simulink model "lyskawaProject_si"  (R2023b)
settings: Solver=VariableStepAuto  StartTime=startTime  StopTime=stopTime  MaxStep=maxStepSize  RelTol=1e-3
values from neighbouring files (symbols this model uses):
  cp = 1000    [lyskawaProject.m]    (also in nieliniowe.m; rStanu.m; test2.m; transmitancje.m)
  Cvp = cp*ro*Vp    (= 18000)    [lyskawaProject.m]    (also in nieliniowe.m; rStanu.m; test2.m = 1500; transmitancje.m)
  Cvw = cp*ro*Vw    (= 36000)    [lyskawaProject.m]    (also in nieliniowe.m; rStanu.m; test2.m = 3000; transmitancje.m)
  dfp = 0    [lyskawaProject.m]    (also in nieliniowe.m = 0.1; rStanu.m; test2.m = 1; transmitancje.m)
  dTk = 0    [lyskawaProject.m]    (also in nieliniowe.m; rStanu.m; transmitancje.m)
  dTz = 5    [lyskawaProject.m]    (also in nieliniowe.m = 0; rStanu.m = 2; transmitancje.m = 2)
  fp0 = fpN    (= 0.47619047619)    [lyskawaProject.m]    (also in nieliniowe.m = vfp0(3); rStanu.m = vfp0(3); test2.m = 0.2; transmitancje.m = vfp0(3))
  K1 = (cp*ro*fpN*(TkN-TpN))/(TwN+2*TpN-3*TzN)    (= 103.896103896)    [lyskawaProject.m]    (also in nieliniowe.m; rStanu.m; test2.m = 275; transmitancje.m)
  K2 = (2*cp*ro*fpN*(TkN - TpN))/(TwN + 2*TpN - 3*TzN)    (= 207.792207792)    [lyskawaProject.m]    (also in nieliniowe.m; rStanu.m; test2.m = 60; transmitancje.m)
  Kp = (2*cp*ro*fpN*(TkN-TpN)*(TpN-TzN))/((TwN-TpN)*(TwN+2*TpN-3*TzN)) -cp*ro*fpN    (= 883.116883117)    [lyskawaProject.m]    (also in nieliniowe.m; rStanu.m; test2.m = 900; transmitancje.m)
  ro = 1.2    [lyskawaProject.m]    (also in nieliniowe.m; rStanu.m; transmitancje.m)
  t0 = 10    [lyskawaProject.m]    (also in nieliniowe.m = 100; rStanu.m = 100; test2.m; transmitancje.m = 100)
  Tk0 = TkN    (= 35)    [lyskawaProject.m]    (also in nieliniowe.m = vTk0(3); rStanu.m = vTk0(3); transmitancje.m = vTk0(3))
  Tp0 = x(2)    [lyskawaProject.m]    (also in nieliniowe.m; rStanu.m; test2.m = 10; transmitancje.m)
  Tw0 = x(1)    [lyskawaProject.m]    (also in nieliniowe.m; rStanu.m; transmitancje.m)
  Tz0 = TzN    (= -20)    [lyskawaProject.m]    (also in nieliniowe.m = vTz0(3); rStanu.m = vTz0(3); transmitancje.m = vTz0(3))
settings Model: Creator=aleklyskawa  LastModifiedBy=aleklyskawa

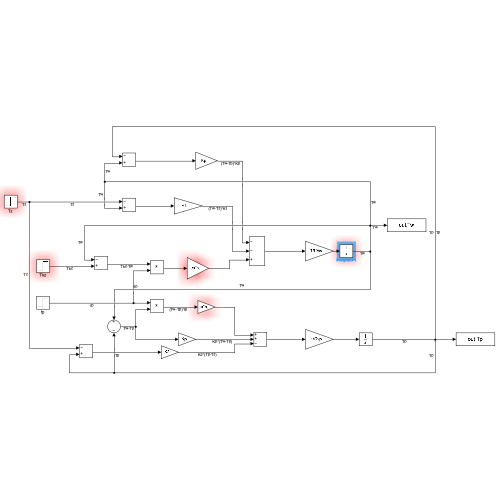
[thumbnail: Simulink's stored preview of the top-level diagram]
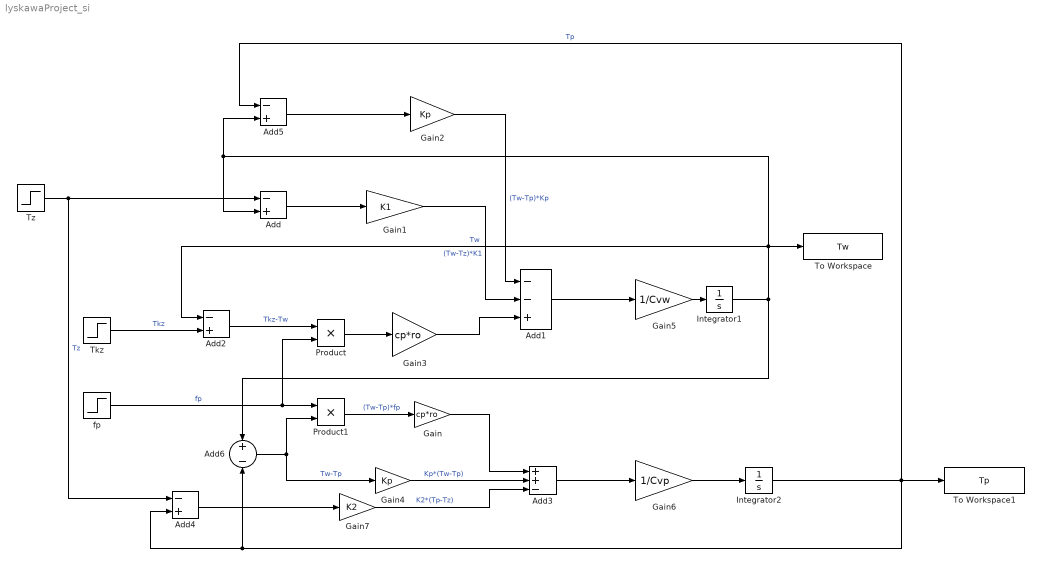
== system lyskawaProject_si ==
  Add{,2,4..5} (4 alike) : Sum  Inputs=-+
  Add1 : Sum  Inputs=--+
  Add3 : Sum  Inputs=++-
  Add6 : Sum  Inputs=+-
  Gain : Gain  Gain=cp*ro
  Gain1 : Gain  Gain=K1
  Gain2 : Gain  Gain=Kp
  Gain3 : Gain  Gain=cp*ro
  Gain4 : Gain  Gain=Kp
  Gain5 : Gain  Gain=1/Cvw
  Gain6 : Gain  Gain=1/Cvp
  Gain7 : Gain  Gain=K2
  Integrator1 : Integrator  InitialCondition=Tw0
  Integrator2 : Integrator  InitialCondition=Tp0
  Product : Product
  Product1 : Product
  Tkz : Step  Time=t0  Before=Tk0  After=Tk0+dTk  SampleTime=0
  To Workspace : ToWorkspace  VariableName=Tw  SampleTime=-1
  To Workspace1 : ToWorkspace  VariableName=Tp  SampleTime=-1
  Tz : Step  Time=t0  Before=Tz0  After=Tz0+dTz  SampleTime=0
  fp : Step  Time=t0  Before=fp0  After=fp0+dfp  SampleTime=0
  wires:
  Tz/1 -> Add4/1, Add/1  "Tz"
  Add/1 -> Gain1/1
  Gain1/1 -> Add1/2  "(Tw-Tz)*K1"
  Add1/1 -> Gain5/1
  Gain5/1 -> Integrator1/1
  Integrator1/1 -> Add5/2, Add/2, To Workspace/1, Add2/1, Add6/1  "Tw"
  Add5/1 -> Gain2/1
  Gain2/1 -> Add1/1  "(Tw-Tp)*Kp"
  Tkz/1 -> Add2/2  "Tkz"
  Add2/1 -> Product/1  "Tkz-Tw"
  Product/1 -> Gain3/1
  Gain3/1 -> Add1/3
  fp/1 -> Product1/1, Product/2  "fp"
  Product1/1 -> Gain/1  "(Tw-Tp)*fp"
  Gain/1 -> Add3/1
  Add6/1 -> Gain4/1, Product1/2  "Tw-Tp"
  Gain4/1 -> Add3/2  "Kp*(Tw-Tp)"
  Add3/1 -> Gain6/1
  Gain6/1 -> Integrator2/1
  Integrator2/1 -> Add5/1, To Workspace1/1, Add6/2, Add4/2  "Tp"
  Add4/1 -> Gain7/1
  Gain7/1 -> Add3/3  "K2*(Tp-Tz)"
